simulink model "DC_Motor"  (R2016a)
settings: Solver=VariableStepAuto  StartTime=0.0  StopTime=3.0  RelTol=1e-3
undefined symbols (not defined in the file): g, G1, G2, J, Ke, Kt, L, l, m, R
settings Model: Creator=mmdclm  LastModifiedBy=Lara

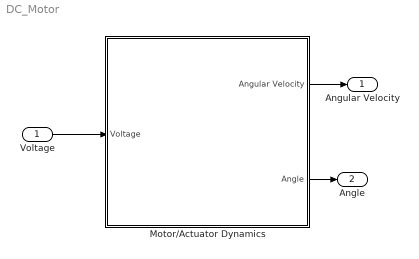
== system DC_Motor ==
  Voltage : Inport
  Motor/Actuator Dynamics : Subsystem
  Angular Velocity : Outport
  Angle : Outport  Port=2
  wires:
  Voltage/1 -> Motor/Actuator Dynamics/1(Voltage)
  Motor/Actuator Dynamics/1(Angular Velocity) -> Angular Velocity/1
  Motor/Actuator Dynamics/2(Angle) -> Angle/1

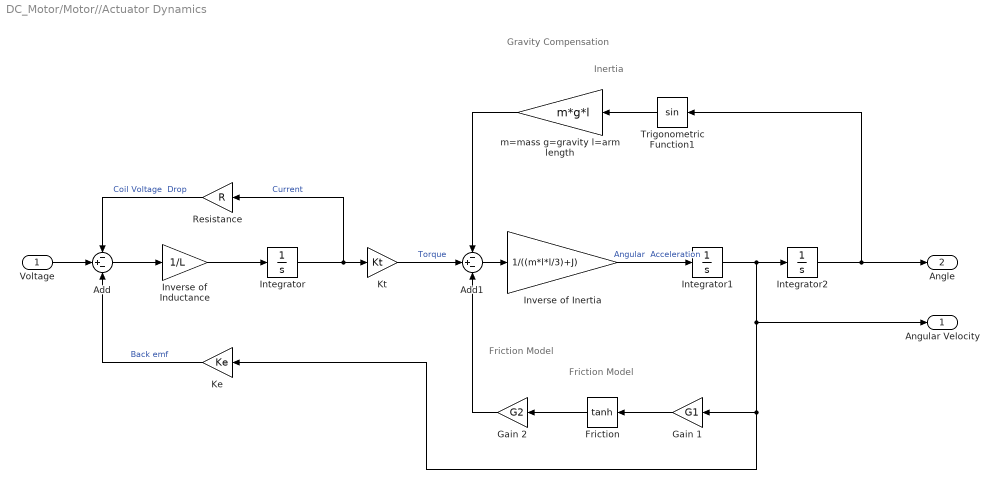
== system DC_Motor/Motor//Actuator Dynamics ==
  note: Friction Model
  note: Gravity Compensation
  note: Inertia
  note: Friction Model
  Voltage : Inport
  Add : Sum  Inputs=-+-
  Add1 : Sum  Inputs=-+-
  "Friction " : Trigonometry  Operator=tanh
  Gain 1 : Gain  Gain=G1
  Gain 2 : Gain  Gain=G2
  Integrator : Integrator
  Integrator1 : Integrator
  Integrator2 : Integrator
  Inverse of Inductance : Gain  Gain=1/L
  "Inverse of Inertia " : Gain  Gain=1/((m*l*l/3)+J)
  "Ke " : Gain  Gain=Ke
  "Kt " : Gain  Gain=Kt
  "Resistance " : Gain  Gain=R
  Trigonometric Function1 : Trigonometry
  m=mass g=gravity l=arm length : Gain  Gain=m*g*l
  Angular Velocity : Outport
  Angle : Outport  Port=2
  wires:
  Voltage/1 -> Add/2
  Inverse of Inductance/1 -> Integrator/1
  Add/1 -> Inverse of Inductance/1
  "Inverse of Inertia "/1 -> Integrator1/1  "Angular  Acceleration"
  "Resistance "/1 -> Add/1  "Coil Voltage  Drop"
  Integrator1/1 -> Angular Velocity/1, "Ke "/1, Gain 1/1, Integrator2/1
  Integrator/1 -> "Kt "/1, "Resistance "/1  "Current"
  "Ke "/1 -> Add/3  "Back emf"
  Gain 1/1 -> "Friction "/1
  "Friction "/1 -> Gain 2/1
  m=mass g=gravity l=arm length/1 -> Add1/1
  Integrator2/1 -> Angle/1, Trigonometric Function1/1
  "Kt "/1 -> Add1/2  "Torque"
  Trigonometric Function1/1 -> m=mass g=gravity l=arm length/1
  Gain 2/1 -> Add1/3
  Add1/1 -> "Inverse of Inertia "/1
